simulink model "InvertedPendulumControl"  (R2017b)
settings: Solver=ode45  StartTime=0.0  StopTime=50  RelTol=1e-9
values from neighbouring files (symbols this model uses):
  B = 1.21e-5    (= 1.21e-05)    [InvertedPendulumMaster.m]
  b = 0.1    [InvertedPendulumMaster.m]
  D = 0    [InvertedPendulumMaster.m]
  g = 9.81    [InvertedPendulumMaster.m]
  I = (1/3)*m*(2*Length)^2    (= 0.00103364533333)    [InvertedPendulumMaster.m]
  J = 2.12e-5    (= 2.12e-05)    [InvertedPendulumMaster.m]
  Kd = 0    [InvertedPendulumMaster.m]
  Kdv = 0    [InvertedPendulumMaster.m]
  Kdx = 0    [InvertedPendulumMaster.m]
  Ki = 0    [InvertedPendulumMaster.m]
  Kiv = 0    [InvertedPendulumMaster.m]
  Kix = 0    [InvertedPendulumMaster.m]
  Kp = 0    [InvertedPendulumMaster.m]
  Kpv = 0    [InvertedPendulumMaster.m]
  Kpx = 0    [InvertedPendulumMaster.m]
  Kt = 0.065    [InvertedPendulumMaster.m]
  Kv = 0.065    [InvertedPendulumMaster.m]
  L = 2.26e-3    (= 0.00226)    [InvertedPendulumMaster.m]
  Length = 0.151    [InvertedPendulumMaster.m]
  M = 0.292    [InvertedPendulumMaster.m]
  m = 0.034    [InvertedPendulumMaster.m]
  R = 1.38    [InvertedPendulumMaster.m]
  r = .0191    (= 0.0191)    [InvertedPendulumMaster.m]
  th0 = 0.05    [InvertedPendulumMaster.m]
  thd0 = 0    [InvertedPendulumMaster.m]
libraries: simulink x3
settings Model: Creator=melab15  LastModifiedBy=journ
settings DataIOCC: TimeSaveName=t
settings DebuggingCC: AlgebraicLoopMsg=none  ArtificialAlgebraicLoopMsg=none
settings CodeAppCC: StateflowObjectComments=on

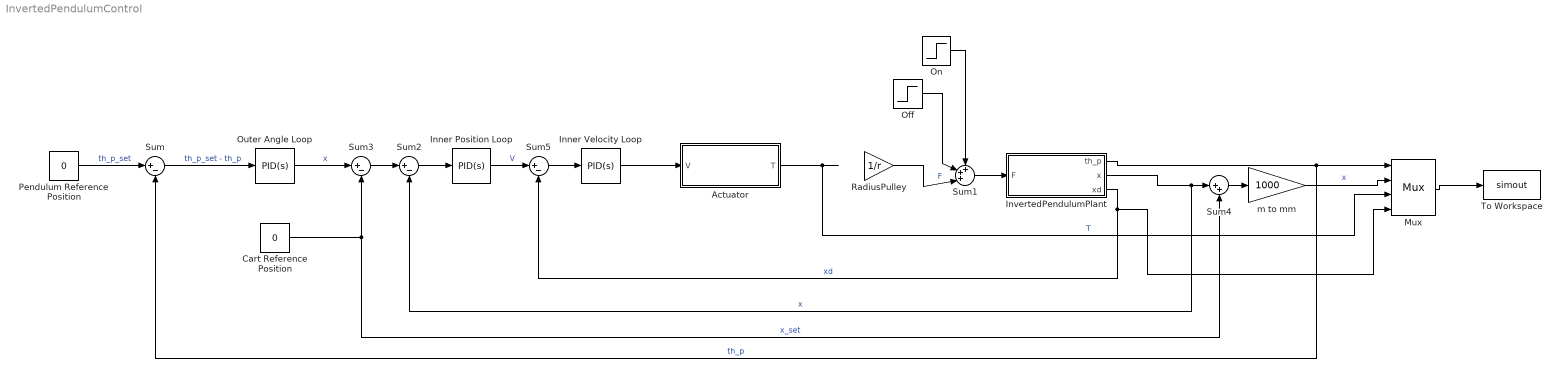
== system InvertedPendulumControl ==
  Actuator : Subsystem
  Cart Reference Position : Constant  Value=0
  Inner Position Loop : simulink/Continuous/PID Controller  Controller=PID  TimeDomain=Continuous-time  SampleTime=-1  IntegratorMethod=Forward Euler  FilterMethod=Forward Euler  Form=Parallel  UseFilter=on  ControllerParametersSource=internal  P=Kpx  I=Kix  D=Kdx  N=100  InitialConditionSource=internal  InitialConditionForIntegrator=0  InitialConditionForFilter=0  ExternalReset=none  LimitOutput=off  UpperSaturationLimit=inf  LowerSaturationLimit=-inf  LinearizeAsGain=on  AntiWindupMode=none  Kb=1  TrackingMode=off  Kt=1  PParamMin=[]  PParamMax=[]  IParamMin=[]  IParamMax=[]  DParamMin=[]  DParamMax=[]  NParamMin=[]  NParamMax=[]  KbParamMin=[]  KbParamMax=[]  KtParamMin=[]  KtParamMax=[]  POutMin=[]  POutMax=[]  IOutMin=[]  IOutMax=[]  DOutMin=[]  DOutMax=[]  NOutMin=[]  NOutMax=[]  KbOutMin=[]  KbOutMax=[]  KtOutMin=[]  KtOutMax=[]  IntegratorOutMin=[]  IntegratorOutMax=[]  FilterOutMin=[]  FilterOutMax=[]  SumOutMin=[]  SumOutMax=[]  SumI1OutMin=[]  SumI1OutMax=[]  SumI2OutMin=[]  SumI2OutMax=[]  SumI3OutMin=[]  SumI3OutMax=[]  SumDOutMin=[]  SumDOutMax=[]  SaturationOutMin=[]  SaturationOutMax=[]  IntegratorContinuousStateAttributes=''  IntegratorStateMustResolveToSignalObject=off  IntegratorRTWStateStorageClass=Auto  FilterContinuousStateAttributes=''  FilterStateMustResolveToSignalObject=off  FilterRTWStateStorageClass=Auto  DifferentiatorICPrevScaledInput=0  DifferentiatorOutMin=[]  DifferentiatorOutMax=[]  InitialConditionSetting=State (most efficient)  FilterDiffOutCoefMin=[]  FilterDiffOutCoefMax=[]  SumDenOutMin=[]  SumDenOutMax=[]  SumNumOutMin=[]  SumNumOutMax=[]  ReciprocalOutMin=[]  ReciprocalOutMax=[]  DivideOutMin=[]  DivideOutMax=[]  TunerSelectOption=Transfer Function Based (PID Tuner App)
  Inner Velocity Loop : simulink/Continuous/PID Controller  Controller=PID  TimeDomain=Continuous-time  SampleTime=-1  IntegratorMethod=Forward Euler  FilterMethod=Forward Euler  Form=Parallel  UseFilter=on  ControllerParametersSource=internal  P=Kpv  I=Kiv  D=Kdv  N=100  InitialConditionSource=internal  InitialConditionForIntegrator=0  InitialConditionForFilter=0  ExternalReset=none  LimitOutput=off  UpperSaturationLimit=inf  LowerSaturationLimit=-inf  LinearizeAsGain=on  AntiWindupMode=none  Kb=1  TrackingMode=off  Kt=1  PParamMin=[]  PParamMax=[]  IParamMin=[]  IParamMax=[]  DParamMin=[]  DParamMax=[]  NParamMin=[]  NParamMax=[]  KbParamMin=[]  KbParamMax=[]  KtParamMin=[]  KtParamMax=[]  POutMin=[]  POutMax=[]  IOutMin=[]  IOutMax=[]  DOutMin=[]  DOutMax=[]  NOutMin=[]  NOutMax=[]  KbOutMin=[]  KbOutMax=[]  KtOutMin=[]  KtOutMax=[]  IntegratorOutMin=[]  IntegratorOutMax=[]  FilterOutMin=[]  FilterOutMax=[]  SumOutMin=[]  SumOutMax=[]  SumI1OutMin=[]  SumI1OutMax=[]  SumI2OutMin=[]  SumI2OutMax=[]  SumI3OutMin=[]  SumI3OutMax=[]  SumDOutMin=[]  SumDOutMax=[]  SaturationOutMin=[]  SaturationOutMax=[]  IntegratorContinuousStateAttributes=''  IntegratorStateMustResolveToSignalObject=off  IntegratorRTWStateStorageClass=Auto  FilterContinuousStateAttributes=''  FilterStateMustResolveToSignalObject=off  FilterRTWStateStorageClass=Auto  DifferentiatorICPrevScaledInput=0  DifferentiatorOutMin=[]  DifferentiatorOutMax=[]  InitialConditionSetting=State (most efficient)  FilterDiffOutCoefMin=[]  FilterDiffOutCoefMax=[]  SumDenOutMin=[]  SumDenOutMax=[]  SumNumOutMin=[]  SumNumOutMax=[]  ReciprocalOutMin=[]  ReciprocalOutMax=[]  DivideOutMin=[]  DivideOutMax=[]  TunerSelectOption=Transfer Function Based (PID Tuner App)
  InvertedPendulumPlant : Subsystem
  Mux : Mux
      settings: DisplayOption=signals
  Off : Step  Time=4.000001  Before=D  After=0  SampleTime=0
  On : Step  Time=4  After=D  SampleTime=0
  Outer Angle Loop : simulink/Continuous/PID Controller  Controller=PID  TimeDomain=Continuous-time  SampleTime=-1  IntegratorMethod=Forward Euler  FilterMethod=Forward Euler  Form=Parallel  UseFilter=on  ControllerParametersSource=internal  P=Kp  I=Ki  D=Kd  N=100  InitialConditionSource=internal  InitialConditionForIntegrator=0  InitialConditionForFilter=0  ExternalReset=none  LimitOutput=off  UpperSaturationLimit=inf  LowerSaturationLimit=-inf  LinearizeAsGain=on  AntiWindupMode=none  Kb=1  TrackingMode=off  Kt=1  PParamMin=[]  PParamMax=[]  IParamMin=[]  IParamMax=[]  DParamMin=[]  DParamMax=[]  NParamMin=[]  NParamMax=[]  KbParamMin=[]  KbParamMax=[]  KtParamMin=[]  KtParamMax=[]  POutMin=[]  POutMax=[]  IOutMin=[]  IOutMax=[]  DOutMin=[]  DOutMax=[]  NOutMin=[]  NOutMax=[]  KbOutMin=[]  KbOutMax=[]  KtOutMin=[]  KtOutMax=[]  IntegratorOutMin=[]  IntegratorOutMax=[]  FilterOutMin=[]  FilterOutMax=[]  SumOutMin=[]  SumOutMax=[]  SumI1OutMin=[]  SumI1OutMax=[]  SumI2OutMin=[]  SumI2OutMax=[]  SumI3OutMin=[]  SumI3OutMax=[]  SumDOutMin=[]  SumDOutMax=[]  SaturationOutMin=[]  SaturationOutMax=[]  IntegratorContinuousStateAttributes=''  IntegratorStateMustResolveToSignalObject=off  IntegratorRTWStateStorageClass=Auto  FilterContinuousStateAttributes=''  FilterStateMustResolveToSignalObject=off  FilterRTWStateStorageClass=Auto  DifferentiatorICPrevScaledInput=0  DifferentiatorOutMin=[]  DifferentiatorOutMax=[]  InitialConditionSetting=State (most efficient)  FilterDiffOutCoefMin=[]  FilterDiffOutCoefMax=[]  SumDenOutMin=[]  SumDenOutMax=[]  SumNumOutMin=[]  SumNumOutMax=[]  ReciprocalOutMin=[]  ReciprocalOutMax=[]  DivideOutMin=[]  DivideOutMax=[]  TunerSelectOption=Transfer Function Based (PID Tuner App)
  Pendulum Reference Position : Constant  Value=0
  RadiusPulley : Gain  Gain=1/r
  Sum{,2..3,5} (4 alike) : Sum  Inputs=|+-
  Sum1 : Sum  Inputs=+++|
  Sum4 : Sum  Inputs=|++
  To Workspace : ToWorkspace  VariableName=simout  SampleTime=-1
  "m to mm " : Gain  Gain=1000
  wires:
  InvertedPendulumPlant/1(th_p) -> Sum/2, Mux/1  "th_p"
  Mux/1 -> To Workspace/1
  "m to mm "/1 -> Mux/2  "x"
  Sum1/1 -> InvertedPendulumPlant/1(F)
  On/1 -> Sum1/1
  Off/1 -> Sum1/2
  Pendulum Reference Position/1 -> Sum/1  "th_p_set"
  Sum/1 -> Outer Angle Loop/1  "th_p_set - th_p"
  RadiusPulley/1 -> Sum1/3  "F"
  Actuator/1(T) -> Mux/3  "T"
  Sum2/1 -> Inner Position Loop/1
  InvertedPendulumPlant/2(x) -> Sum4/1, Sum2/2  "x"
  Sum3/1 -> Sum2/1
  Outer Angle Loop/1 -> Sum3/1  "x"
  Sum4/1 -> "m to mm "/1
  Cart Reference Position/1 -> Sum4/2, Sum3/2  "x_set"
  Sum5/1 -> Inner Velocity Loop/1
  Inner Position Loop/1 -> Sum5/1  "V"
  Inner Velocity Loop/1 -> Actuator/1(V)
  InvertedPendulumPlant/3(xd) -> Mux/4, Sum5/2  "xd"

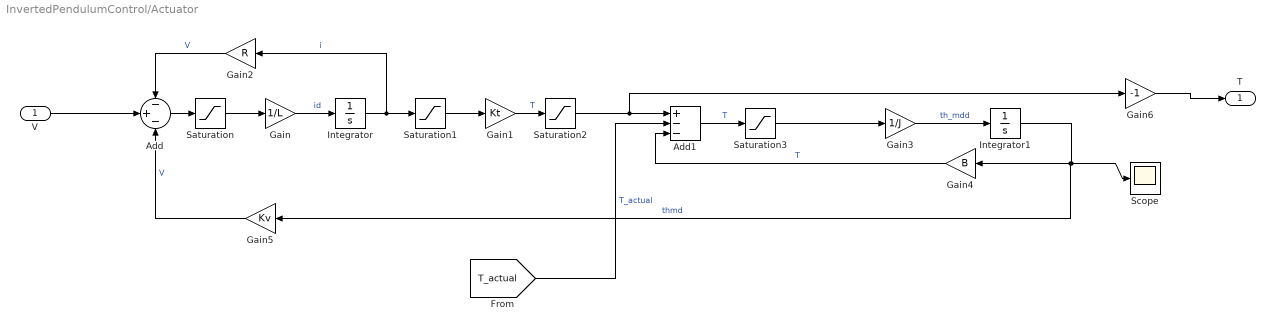
== system InvertedPendulumControl/Actuator ==
  V : Inport
  Add : Sum  Inputs=-+-
  Add1 : Sum  Inputs=+--
  Gain : Gain  Gain=1/L
  Gain1 : Gain  Gain=Kt
  Gain2 : Gain  Gain=R
  Gain3 : Gain  Gain=1/J
  Gain4 : Gain  Gain=B
  Gain5 : Gain  Gain=Kv
  Gain6 : Gain  Gain=-1
  Integrator : Integrator
  Integrator1 : Integrator
  Saturation : Saturate  UpperLimit=24  LowerLimit=-24
  Saturation1 : Saturate  UpperLimit=17.4  LowerLimit=-17.4
  Saturation2 : Saturate  UpperLimit=1.225  LowerLimit=-1.225
  Saturation3 : Saturate  UpperLimit=1.225  LowerLimit=-1.225
  Scope : Scope
  T : Outport
  wires:
  V/1 -> Add/2
  Add/1 -> Saturation/1
  Gain/1 -> Integrator/1  "id"
  Integrator/1 -> Gain2/1, Saturation1/1  "i"
  Gain2/1 -> Add/1  "V"
  Gain3/1 -> Integrator1/1  "th_mdd"
  Integrator1/1 -> Scope/1, Gain5/1, Gain4/1  "thmd"
  Gain4/1 -> Add1/3  "T"
  Gain5/1 -> Add/3  "V"
  Add1/1 -> Saturation3/1  "T"
  [T_actual] -> Add1/2  "T_actual"
  Gain1/1 -> Saturation2/1  "T"
  Saturation/1 -> Gain/1
  Saturation1/1 -> Gain1/1
  Saturation2/1 -> Gain6/1, Add1/1
  Saturation3/1 -> Gain3/1
  Gain6/1 -> T/1

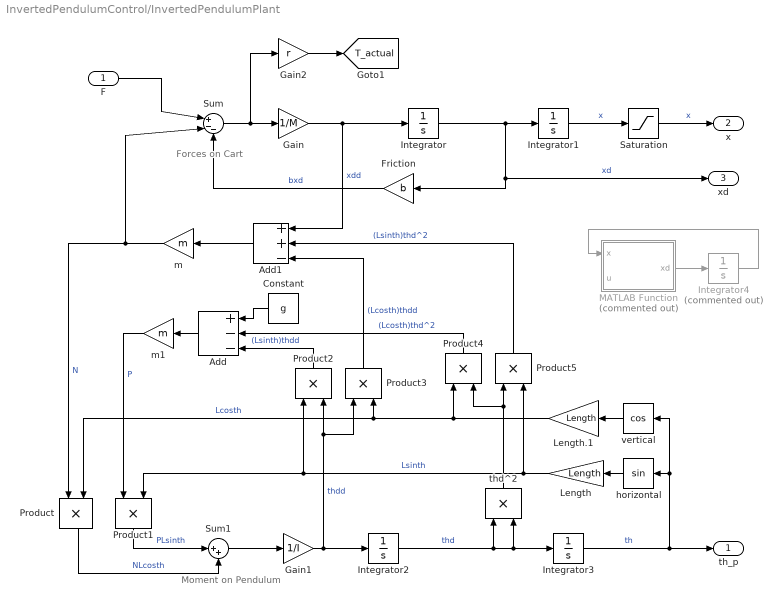
== system InvertedPendulumControl/InvertedPendulumPlant ==
  note: Forces on Cart
  note: Moment on Pendulum
  F : Inport
  Add : Sum  Inputs=+--
  Add1 : Sum  Inputs=++-
  Constant : Constant  Value=g
  Friction : Gain  Gain=b
  Gain : Gain  Gain=1/M
  Gain1 : Gain  Gain=1/I
  Gain2 : Gain  Gain=r
  Integrator : Integrator
  Integrator1 : Integrator
  Integrator2 : Integrator  InitialCondition=thd0
  Integrator3 : Integrator  InitialCondition=th0
  Integrator4 : Integrator  Commented=on
  Length : Gain  Gain=Length
  Length.1 : Gain  Gain=Length
  MATLAB Function : MATLAB Function  Commented=on  TreatAsAtomicUnit=on
  Product{,1..5} (6 alike) : Product
  Saturation : Saturate  UpperLimit=0.2413  LowerLimit=-0.2413
  Sum : Sum  Inputs=|+--
  Sum1 : Sum  Inputs=|++
  horizontal : Trigonometry
  m : Gain  Gain=m
  m1 : Gain  Gain=m
  thd^2 : Product
  "vertical " : Trigonometry  Operator=cos
  th_p : Outport
  x : Outport  Port=2
  xd : Outport  Port=3
  tag scope: T_actual=global
  wires:
  Gain/1 -> Add1/1, Integrator/1  "xdd"
  Product3/1 -> Add1/3  "(Lcosth)thdd"
  Length.1/1 -> Product4/1, Product3/2, Product/2  "Lcosth"
  Constant/1 -> Add/1
  Add/1 -> m1/1
  Product2/1 -> Add/3  "(Lsinth)thdd"
  Integrator3/1 -> th_p/1, "vertical "/1, horizontal/1  "th"
  Product/1 -> Sum1/2  "NLcosth"
  horizontal/1 -> Length/1
  Product5/1 -> Add1/2  "(Lsinth)thd^2"
  Sum/1 -> Gain2/1, Gain/1
  Friction/1 -> Sum/3  "bxd"
  thd^2/1 -> Product4/2, Product5/1
  m1/1 -> Product1/1  "P"
  Product1/1 -> Sum1/1  "PLsinth"
  Add1/1 -> m/1
  Product4/1 -> Add/2  "(Lcosth)thd^2"
  Integrator2/1 -> thd^2/1, thd^2/2, Integrator3/1  "thd"
  Gain1/1 -> Product3/1, Product2/2, Integrator2/1  "thdd"
  Sum1/1 -> Gain1/1
  Length/1 -> Product5/2, Product2/1, Product1/2  "Lsinth"
  Integrator/1 -> Friction/1, xd/1, Integrator1/1  "xd"
  m/1 -> Sum/2, Product/1  "N"
  "vertical "/1 -> Length.1/1
  Saturation/1 -> x/1  "x"
  MATLAB Function/1(xd) -> Integrator4/1
  Integrator4/1 -> MATLAB Function/1(x)
  Gain2/1 -> [T_actual]
  Integrator1/1 -> Saturation/1  "x"
  F/1 -> Sum/1

== matlab function InvertedPendulumControl/InvertedPendulumPlant/MATLAB Function ==
  data: x input; u input; xd output
function xd  = nonlinSS(x,u)

xd = u + x;
